simulink model "RB_dyn"  (R2024b)
settings: Solver=ode15s  StartTime=0.0  StopTime=50  RelTol=1e-4
model workspace (MAT data in the model file):
  op_trim1 : opcond.OperatingReport (value not decoded)
  op_trim2 : opcond.OperatingReport (value not decoded)
  op_trim3 : opcond.OperatingReport (value not decoded)
values from neighbouring files (symbols this model uses):
  B_p = 1/(m_t_est)    [MAIN_exam_2025.m]
  F_matrix = zeros(6, 6)    [MAIN_exam_2025.m]
  Finv = pinv(F_matrix)    [MAIN_exam_2025.m]
  GAMMA_a = diag([0.5, 0.5, 0.5,1, 1, 1, 1, 1, 1, 1])    [MAIN_exam_2025.m]
  k_f = 3.65e-6    (= 3.65e-06)    [MAIN_exam_2025.m]
  K_position = diag([K_px, K_py, K_pz])    [MAIN_exam_2025.m]
  Ki = diag([K_ix, K_iy, K_iz])    [MAIN_exam_2025.m]
  Kp = diag([K_dx, K_dy, K_dz])    [MAIN_exam_2025.m]
  L = 100    [MAIN_exam_2025.m]
  LAMBDA_hat_0 = ones(3,1)    [MAIN_exam_2025.m]
  Lambda_matrix = diag([1, 1, 1, 1,1, 1])    [MAIN_exam_2025.m]
  m_t_est = UAV.m0 + m_p    [MAIN_exam_2025.m]
  omegab_0 = [0 0 0]'    [MAIN_exam_2025.m]
  p_0 = [-24 8 2.5]'    [MAIN_exam_2025.m]
  p_x_data = p_lookup(:,1)    [MAIN_exam_2025.m]
  p_y_data = p_lookup(:,2)    [MAIN_exam_2025.m]
  p_z_data = p_lookup(:,3)    [MAIN_exam_2025.m]
  q_0 = eul2quat([0, 0, 0 ]*degToRad,'XYZ')'    [MAIN_exam_2025.m]
  t_lookup = ts_pos.Time    [MAIN_exam_2025.m]
  Theta_0 = [0;0;(m_t_est)*par.g;D_fv_bar(1,1);D_fv_bar(2,2);D_fv_bar(3,3)]    [MAIN_exam_2025.m]
  v_0 = R_0*vb_0    [MAIN_exam_2025.m]
  vb_0 = [0 0 0]'    [MAIN_exam_2025.m]
undefined symbols (not defined in the file or in its folder): ctrl, par, proj, UAV
(part 2 of 2)

== matlab function RB_dyn/Predictor/Adaptive Laws/Projection and integration 1/Projection Dz/Projection ==
  data: theta input; y_proj output; y input; GAMMA_a parameter; proj parameter
function y_proj = proj(theta,y,GAMMA_a, proj)
Gamma = GAMMA_a(9,9);
eps_proj = proj.eps;
theta_M = proj.RDz;
center = proj.CenterDz;
theta = theta - center;

f = 1/(eps_proj*theta_M^2)*((1+eps_proj)*(theta')*theta-theta_M^2);
grad_f = 2/(eps_proj*theta_M^2)*(1+eps_proj)*theta;

if f>0 && y'*Gamma*grad_f>0
    y_proj = Gamma*y - f*Gamma*(grad_f)*grad_f'/(grad_f'*Gamma*grad_f)*Gamma*y;
else
    y_proj = Gamma*y;
  
end

== matlab function RB_dyn/Predictor/Adaptive Laws/Projection and integration 1/Projection lambda1/Projection ==
  data: theta input; y_proj output; y input; GAMMA_a parameter; proj parameter
function y_proj = proj(theta,y,GAMMA_a, proj)
Gamma = GAMMA_a(1,1);
eps_proj = proj.eps;
theta_M = proj.RLambda;
center = proj.CenterLambda;
theta = theta - center;

f = 1/(eps_proj*theta_M^2)*((1+eps_proj)*(theta')*theta-theta_M^2);
grad_f = 2/(eps_proj*theta_M^2)*(1+eps_proj)*theta;

if f>0 && y'*Gamma*grad_f>0
    y_proj = Gamma*y - f*Gamma*(grad_f)*grad_f'/(grad_f'*Gamma*grad_f)*Gamma*y;
else
    y_proj = Gamma*y;
  
end

== matlab function RB_dyn/Predictor/Adaptive Laws/Projection and integration 1/Projection lambda2/Projection ==
  data: theta input; y_proj output; y input; GAMMA_a parameter; proj parameter
function y_proj = proj(theta,y,GAMMA_a, proj)
Gamma = GAMMA_a(2,2);
eps_proj = proj.eps;
theta_M = proj.RLambda;
center = proj.CenterLambda;
theta = theta - center;

f = 1/(eps_proj*theta_M^2)*((1+eps_proj)*(theta')*theta-theta_M^2);
grad_f = 2/(eps_proj*theta_M^2)*(1+eps_proj)*theta;

if f>0 && y'*Gamma*grad_f>0
    y_proj = Gamma*y - f*Gamma*(grad_f)*grad_f'/(grad_f'*Gamma*grad_f)*Gamma*y;
else
    y_proj = Gamma*y;
  
end

== matlab function RB_dyn/Predictor/Adaptive Laws/Projection and integration 1/Projection lambda3/Projection ==
  data: theta input; y_proj output; y input; GAMMA_a parameter; proj parameter
function y_proj = proj(theta,y,GAMMA_a, proj)
Gamma = GAMMA_a(3,3);
eps_proj = proj.eps;
theta_M = proj.RLambda;
center = proj.CenterLambda;
theta = theta - center;

f = 1/(eps_proj*theta_M^2)*((1+eps_proj)*(theta')*theta-theta_M^2);
grad_f = 2/(eps_proj*theta_M^2)*(1+eps_proj)*theta;

if f>0 && y'*Gamma*grad_f>0
    y_proj = Gamma*y - f*Gamma*(grad_f)*grad_f'/(grad_f'*Gamma*grad_f)*Gamma*y;
else
    y_proj = Gamma*y;
  
end

== matlab function RB_dyn/MATLAB Function1 ==
  data: p_r input; alpha output; p_d input
function alpha = fcn(p_r, p_d)

error = norm(p_r-p_d);
alpha = 1 / (1 + 0.05* error^2);

== matlab function RB_dyn/Dinámica UAV/Rigid Body dynamics&kinematics /MATLAB Function3 ==
  data: q input; R output
function R = fcn(q)

R = quat2rotm(q');

end

== matlab function RB_dyn/Atittude Planner & Controller/Atittude Controller/Geodesian error1 ==
  data: E output; Rd input; R input
function E = error(Rd, R)
    % Parámetros de ganancia (ajustables)
    % k_tp: importancia de mantener el eje de empuje (evitar caerse)
    % k_psi: importancia de mirar hacia el frente (yaw)
    k_tp = 1.0; 
    k_psi = 0.2; 

    % Extraemos los vectores columna de las matrices de rotación
    % Rd = [iD, jD, kD] | R = [iB, jB, kB]
    iD = Rd(:, 1); jD = Rd(:, 2); kD = Rd(:, 3);
    iB =  R(:, 1); jB =  R(:, 2); kB =  R(:, 3);

    % 1. Error de inclinación (Thrust axis tracking)
    % Se calcula mediante el producto vectorial entre el eje Z deseado y el real
    % Esto busca el camino más corto (geodésica) en la esfera
    e_tilt = cross(kD, kB);

    % 2. Error de encabezado (Heading tracking)
    % Este término desacopla el yaw del eje de empuje
    e_heading = (1/2) * (dot(jD, iB) - dot(iD, jB)) * kB;

    % 3. Error de actitud total (en coordenadas globales/cuerpo según tu control)
    % e_R_tp = k_theta_phi * (kD x kB) + (k_psi/2) * (jD'*iB - iD'*jB) * kB
    E = k_tp * e_tilt + k_psi * e_heading;
end

== matlab function RB_dyn/Dinámica UAV/MATLAB Function ==
  data: p_i input; vw output; wind parameter
function vw = fcn(p_i, wind)

pix = p_i(1);
w = wind(1);
if pix <-21.8
    vw_i = w;
elseif pix> -2 && pix < 3.6
        vw_i = w;
elseif pix>18.8
    vw_i = w;
else
    vw_i = wind(2);
end
vw = [0;vw_i;0];

== matlab function RB_dyn/Dinámica UAV/Rigid Body dynamics&kinematics /MATLAB Function4 ==
  data: a input; c output; b input
function c = cross_six(a,b)

a_v = a(1:3);
a_omega = a(4:6);

cross_six = [crossmat(a_omega), zeros(3,3);
             crossmat(a_v), crossmat(a_omega)] ;

c = cross_six*b;

end

function S=crossmat(s)
S=[0  -s(3)  s(2);
    s(3)   0 -s(1);
    -s(2)  s(1)  0];
end

== matlab function RB_dyn/Dinámica UAV/Gravity wrench ==
  data: R input; w_g output; UAV parameter; par parameter
function w_g = fcn(R,UAV,par)

e_3 = par.e_3;
g = par.g;

w_g = g*[UAV.m*R'*e_3; UAV.S*R'*e_3];

== matlab function RB_dyn/Dinámica UAV/Aerodynamic Damping ==
  data: v_b input; D output; omega_b input; UAV parameter; vw input
function D = Aero(v_b, omega_b, UAV, vw)

D = zeros(6,1);
D = UAV.D*[(v_b - vw);omega_b];

== matlab function RB_dyn/Predictor/Diag ==
  data: u input; y output
function y = fcn(u)

y = diag(u);

== matlab function RB_dyn/Atittude Planner & Controller/Atittude Planner/MATLAB Function ==
  data: fc input; kp output
function kp = kp_fnc(fc)

kp = fc/norm(fc);

== matlab function RB_dyn/Atittude Planner & Controller/Atittude Planner/MATLAB Function1 ==
  settings: updateMethod=DISCRETE
  data: hd output; psi_d input
function hd = header(psi_d)

hd = [cos(psi_d);sin(psi_d);0];

end

== matlab function RB_dyn/Atittude Planner & Controller/Atittude Planner/MATLAB Function2 ==
  data: ip output; kp input; jp output; hd input
function [ip, jp] = y_axis(kp, hd)
    % 1. Aseguramos columnas (aunque el reporte diga que ya lo son)
    kp = kp(:);
    hd = hd(:);

    % 2. PRODUCTO VECTORIAL MANUAL (Sustituye a cross(kp, hd))
    % Matemáticamente: [ y1*z2 - z1*y2; ... ]
    jp_raw = [ kp(2)*hd(3) - kp(3)*hd(2); ...
               kp(3)*hd(1) - kp(1)*hd(3); ...
               kp(1)*hd(2) - kp(2)*hd(1) ];

    % 3. Normalización y protección
    norma = norm(jp_raw);
    if norma < 1e-6
        jp = [0; 1; 0]; 
    else
        jp = jp_raw / norma;
    end
    
    % 4. SEGUNDO PRODUCTO VECTORIAL MANUAL (Sustituye a cross(jp, kp))
    ip = [ jp(2)*kp(3) - jp(3)*kp(2); ...
           jp(3)*kp(1) - jp(1)*kp(3); ...
           jp(1)*kp(2) - jp(2)*kp(1) ];
end

== matlab function RB_dyn/Allocation + Actuator Dynamics/Actuator Dynamics/Thrust Model /Dinamica ==
  data: Omegas input; T_arg output; k_f parameter
function T_arg = fcn(Omegas, k_f)

T_arg = k_f*Omegas.^2;
